simulink model "Week2_Sum4"  (R2020b)
settings: Solver=ode14x  StartTime=0.0  StopTime=5  FixedStep=0.1  RelTol=1e-3
PreLoadFcn:
  | clc;
  | clear all;
  | close all;
  | R = 4;
  | L = 2.75E-6;
  | K = 0.0274;
  | J = 3.2284E-6;
  | b = 3.5077E-6;
settings Model: DataDictionary=Datad1.sldd  Creator=Aradhana desai  LastModifiedBy=Aradhana desai

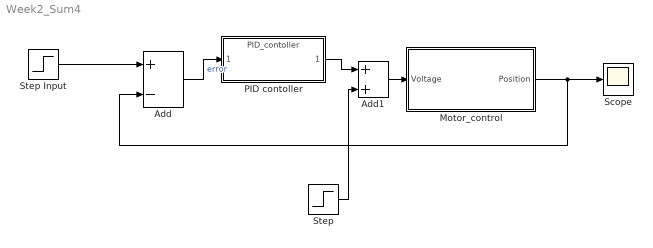
== system Week2_Sum4 ==
  Add : Sum  Inputs=+-
  Add1 : Sum
  Motor_control : Subsystem
  PID contoller : ModelReference  ModelNameDialog=PID_contoller  SimulationMode=Normal  ModelReferenceVersion=1.22
  Scope : Scope
  Step : Step  Time=0  SampleTime=0
  Step Input : Step  Time=0  SampleTime=0
  wires:
  PID contoller/1 -> Add1/1
  Motor_control/1(Position) -> Add/2, Scope/1
  Add/1 -> PID contoller/1  "error"
  Step Input/1 -> Add/1
  Add1/1 -> Motor_control/1(Voltage)
  Step/1 -> Add1/2

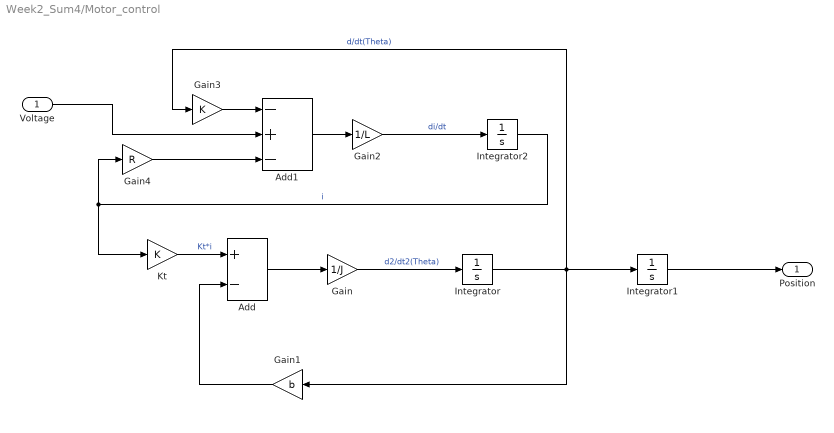
== system Week2_Sum4/Motor_control ==
  Voltage : Inport
  Add : Sum  Inputs=+-
  Add1 : Sum  Inputs=-+-
  Gain : Gain  Gain=1/J
  Gain1 : Gain  Gain=b
  Gain2 : Gain  Gain=1/L
  Gain3 : Gain  Gain=K
  Gain4 : Gain  Gain=R
  Integrator : Integrator
  Integrator1 : Integrator
  Integrator2 : Integrator
  Kt : Gain  Gain=K
  Position : Outport
  wires:
  Gain1/1 -> Add/2
  Integrator2/1 -> Gain4/1, Kt/1  "i"
  Add/1 -> Gain/1
  Integrator/1 -> Gain3/1, Gain1/1, Integrator1/1  "d/dt(Theta)"
  Gain3/1 -> Add1/1
  Gain/1 -> Integrator/1  "d2/dt2(Theta)"
  Gain4/1 -> Add1/3
  Add1/1 -> Gain2/1
  Kt/1 -> Add/1  "Kt*i"
  Gain2/1 -> Integrator2/1  "di/dt"
  Voltage/1 -> Add1/2
  Integrator1/1 -> Position/1
